simulink library "LopesDevelopmentLibrary"  (R2015b)
settings: Solver=ode45  StartTime=0.0  StopTime=10.0  RelTol=1e-3
values from neighbouring files (symbols this model uses):
  d2r = @(d) d*(pi/180)    [LopesDevelopmentLibrary_LoadParameters.m]
  ts = LopesParams.ts    [LopesDevelopmentLibrary_LoadParameters.m]
undefined symbols (not defined in the file or in its folder): anyParameterChanged, DiscIntNeverNeededParam, gcbh, LAP, LHF, LKF, LopesParams, macaddr, mxpcnetworkconfig, mxpcrtudprx, mxpcrtudptx, patientParametersChanged, port, PX, PZ, RAP, RHF, RKF, SelectorLOPESInSize, StrideTime_s, Time
undefined symbols (not defined in the file): LopesParamsSendDataArrayLen
libraries: LopesDevelopmentLibrary x327, simulink x100, dspmtrx3 x49, xpciplib x6, xpcnetworkbufferlib x5, dspsigops x4, dspstat3 x3, xpcethernetlib x2, visionstatistics x2, xpcseriallib x2, LopesDevelopmentLibraryTest x1, nmc x1
(part 3 of 12)

== system LopesDevelopmentLibrary/StringFunctions/Pad ==
  s : Inport
  pad : MATLAB Function  TreatAsAtomicUnit=on
  y : Outport
  y_len : Outport  Port=2
  wires:
  pad/1(y) -> y/1
  s/1 -> pad/1(s)
  pad/2(y_len) -> y_len/1

== system LopesDevelopmentLibrary/StringFunctions/PadStrAsDouble ==
  note: This block pads a string array; the output is as an array of doubles
      | (needed for exception blocks).
  s : Inport
  Data Type Conversion : DataTypeConversion  OutDataTypeStr=double
  pad : MATLAB Function  TreatAsAtomicUnit=on
  y : Outport
  y_len : Outport  Port=2
  wires:
  Data Type Conversion/1 -> y/1
  pad/1(y) -> Data Type Conversion/1
  s/1 -> pad/1(s)
  pad/2(y_len) -> y_len/1

== system LopesDevelopmentLibrary/StringFunctions/concat5 ==
  s1 : Inport
  s1_len : Inport  Port=2
  s2 : Inport  Port=3
  s2_len : Inport  Port=4
  s3 : Inport  Port=5
  s3_len : Inport  Port=6
  s4 : Inport  Port=7
  s4_len : Inport  Port=8
  s5 : Inport  Port=9
  s5_len : Inport  Port=10
  concat5 : MATLAB Function  TreatAsAtomicUnit=on
  str : Outport
  strLen : Outport  Port=2
  wires:
  s5_len/1 -> concat5/10(s5_len)
  s3_len/1 -> concat5/6(s3_len)
  s3/1 -> concat5/5(s3)
  concat5/1(y) -> str/1
  s1_len/1 -> concat5/2(s1_len)
  s2/1 -> concat5/3(s2)
  s4/1 -> concat5/7(s4)
  s2_len/1 -> concat5/4(s2_len)
  s4_len/1 -> concat5/8(s4_len)
  s5/1 -> concat5/9(s5)
  s1/1 -> concat5/1(s1)
  concat5/2(y_len) -> strLen/1

== system LopesDevelopmentLibrary/Various/AddToMatrixColumn ==
  A : Inport
  V : Inport  Port=2
  Maximum : Constant  Value=maximum
  Minimum : Constant  Value=minimum
  Overwrite Values : dspmtrx3/Overwrite Values  OverWriteDiag=Submatrix  valFrom2ndIP=Second input port  ConstValue=0  RowSpan=All rows  RowStartMode=Index  RowStartIndex=row  RowEndMode=Last  RowEndIndex=1  ColSpan=One column  ColStartMode=Index  ColStartIndex=col  ColEndMode=Last  ColEndIndex=1  DiagSpan=Range of elements  DiagStartMode=Index  DiagStartIndex=2  DiagEndMode=Index  DiagEndIndex=4
  Saturation Dynamic : simulink/Discontinuities/Saturation Dynamic  OutMin=[]  OutMax=[]  OutDataTypeStr=Inherit: Same as second input  OutDataType=fixdt(1, 16)  OutScaling=2^-10  DoSatur=off
  Submatrix : dspmtrx3/Submatrix  RowSpan=All rows  RowStartMode=Index  RowStartIndex=row  RowEndMode=Index  RowEndIndex=1  ColSpan=One column  ColStartMode=Index  ColStartIndex=col  ColEndMode=Last  ColEndIndex=1
  Sum : Sum  Inputs=|++
  B : Outport
  wires:
  Minimum/1 -> Saturation Dynamic/3
  Maximum/1 -> Saturation Dynamic/1
  Saturation Dynamic/1 -> Overwrite Values/2
  Sum/1 -> Saturation Dynamic/2
  A/1 -> Submatrix/1, Overwrite Values/1
  Overwrite Values/1 -> B/1
  Submatrix/1 -> Sum/1
  V/1 -> Sum/2

== system LopesDevelopmentLibrary/Various/AddToMatrixElement ==
  A : Inport
  V : Inport  Port=2
  Maximum : Constant  Value=maximum
  Minimum : Constant  Value=minimum
  Overwrite Values : dspmtrx3/Overwrite Values  OverWriteDiag=Submatrix  valFrom2ndIP=Second input port  ConstValue=0  RowSpan=One row  RowStartMode=Index  RowStartIndex=row  RowEndMode=Last  RowEndIndex=1  ColSpan=One column  ColStartMode=Index  ColStartIndex=col  ColEndMode=Last  ColEndIndex=1  DiagSpan=Range of elements  DiagStartMode=Index  DiagStartIndex=2  DiagEndMode=Index  DiagEndIndex=4
  Saturation Dynamic : simulink/Discontinuities/Saturation Dynamic  OutMin=[]  OutMax=[]  OutDataTypeStr=Inherit: Same as second input  OutDataType=fixdt(1, 16)  OutScaling=2^-10  DoSatur=off
  Submatrix : dspmtrx3/Submatrix  RowSpan=One row  RowStartMode=Index  RowStartIndex=row  RowEndMode=Index  RowEndIndex=1  ColSpan=One column  ColStartMode=Index  ColStartIndex=col  ColEndMode=Last  ColEndIndex=1
  Sum : Sum  Inputs=|++
  B : Outport
  wires:
  V/1 -> Sum/2
  Submatrix/1 -> Sum/1
  Overwrite Values/1 -> B/1
  A/1 -> Overwrite Values/1, Submatrix/1
  Sum/1 -> Saturation Dynamic/2
  Saturation Dynamic/1 -> Overwrite Values/2
  Maximum/1 -> Saturation Dynamic/1
  Minimum/1 -> Saturation Dynamic/3

== system LopesDevelopmentLibrary/Various/AdjustAmplitude ==
  note: This block multiplies all positions, velocities and accelerations by input V;
      | in other words,  it just scales the amplitude of the total curve.
  M : Inport
  V : Inport  Port=2
  Matrix Concatenate : Concatenate  Mode=Multidimensional array  ConcatenateDimension=2
  Product : Product  RndMeth=Zero
  angle_vel_acc : dspmtrx3/Submatrix  RowSpan=All rows  RowStartMode=First  RowStartIndex=1  RowEndMode=Last  RowEndIndex=1  ColSpan=Range of columns  ColStartMode=Index  ColStartIndex=2  ColEndMode=Last  ColEndIndex=1
  times : dspmtrx3/Submatrix  RowSpan=All rows  RowStartMode=First  RowStartIndex=1  RowEndMode=Last  RowEndIndex=1  ColSpan=One column  ColStartMode=First  ColStartIndex=1  ColEndMode=Last  ColEndIndex=1
  Y : Outport
  wires:
  Product/1 -> Matrix Concatenate/2
  times/1 -> Matrix Concatenate/1
  angle_vel_acc/1 -> Product/1
  Matrix Concatenate/1 -> Y/1
  M/1 -> times/1, angle_vel_acc/1
  V/1 -> Product/2

== system LopesDevelopmentLibrary/Various/AnyChanged ==
  note: Outputs true if any of the bus elements of the inputs changed during this sample.
  BusIn : Inport
  Bus to Vector : BusToVector
  Detect Change : simulink/Logic and Bit Operations/Detect Change  vinit=0  InputProcessing=Inherited  OutDataTypeStr=boolean
  Logical Operator : Logic  Operator=OR  Inputs=1  AllPortsSameDT=off  OutDataTypeStr=boolean
  Changed : Outport
  wires:
  Bus to Vector/1 -> Detect Change/1
  Detect Change/1 -> Logical Operator/1
  BusIn/1 -> Bus to Vector/1
  Logical Operator/1 -> Changed/1

== system LopesDevelopmentLibrary/Various/AssignMatrixElement ==
  A : Inport
  V : Inport  Port=2
  Maximum : Constant  Value=maximum
  Minimum : Constant  Value=minimum
  Overwrite Values : dspmtrx3/Overwrite Values  OverWriteDiag=Submatrix  valFrom2ndIP=Second input port  ConstValue=0  RowSpan=One row  RowStartMode=Index  RowStartIndex=row  RowEndMode=Last  RowEndIndex=1  ColSpan=One column  ColStartMode=Index  ColStartIndex=col  ColEndMode=Last  ColEndIndex=1  DiagSpan=Range of elements  DiagStartMode=Index  DiagStartIndex=2  DiagEndMode=Index  DiagEndIndex=4
  Saturation Dynamic : simulink/Discontinuities/Saturation Dynamic  OutMin=[]  OutMax=[]  OutDataTypeStr=Inherit: Same as second input  OutDataType=fixdt(1, 16)  OutScaling=2^-10  DoSatur=off
  B : Outport
  wires:
  Minimum/1 -> Saturation Dynamic/3
  Maximum/1 -> Saturation Dynamic/1
  Saturation Dynamic/1 -> Overwrite Values/2
  V/1 -> Saturation Dynamic/2
  Overwrite Values/1 -> B/1
  A/1 -> Overwrite Values/1

== system LopesDevelopmentLibrary/Various/BetterSpringVelocities ==
  note: If you happen to have the analytical accelerations of the spring positions,
      | you can slightly improve the performance of the system by incorporating them
      | in the velocitiy term. The idea is that the SpringVelocities_in reflect the velocity
      | at (discrete) time t=k, but they will be used throughout the sample, thus  during k<=t<k+1.
      | It would be more accurate to use the velocity halfway that period, i.e. at t=k+0.5. The best
      | estimate of that velocity we can get is by doing first order extrapolation, by using the acceleration.
      | Using Forwarrd Euler, we find v_{k+0.5} = v_k + a_k *0.5*ts, with ts the sample time.
  SpringVelocities_in : Inport
  SpringAccelerations_in : Inport  Port=2
  Add1 : Sum
  EnableAccelerationOptimization : Constant  OutDataTypeStr=double
      settings: OpenFcn=|
      | b = get_param(gcb,'value');
      | if (strcmp(b,'1')),
      |   set_param (gcb,'value','0');
      | else
      |   set_param(gcb,'value','1');
      | end;
  Half : Gain  Gain=0.5
  Product : Product  RndMeth=Zero
  SampleTimeGain : Gain  Gain=LopesParams.ts
  SpringVelocities_out : Outport
  wires:
  EnableAccelerationOptimization/1 -> Product/2
  SampleTimeGain/1 -> Half/1
  SpringAccelerations_in/1 -> SampleTimeGain/1
  Product/1 -> Add1/2
  SpringVelocities_in/1 -> Add1/1
  Add1/1 -> SpringVelocities_out/1
  Half/1 -> Product/1

== system LopesDevelopmentLibrary/Various/CompareAny ==
  In1 : Inport
  Compare To Constant : simulink/Logic and Bit Operations/Compare To Constant  relop===  const=values  OutDataTypeStr=boolean
  Logical Operator : Logic  Operator=OR  Inputs=1  AllPortsSameDT=off  OutDataTypeStr=boolean
  Out1 : Outport
  wires:
  Logical Operator/1 -> Out1/1
  Compare To Constant/1 -> Logical Operator/1
  In1/1 -> Compare To Constant/1

== system LopesDevelopmentLibrary/Various/CrossFade ==
  In1 : Inport
  In2 : Inport  Port=2
  AmountIn2 : Inport  Port=3
  Add : Sum  Inputs=+-
  Add1 : Sum
  One : Constant
  Product : Product  RndMeth=Zero
  Product1 : Product  RndMeth=Zero
  Saturation : Saturate  UpperLimit=1  LowerLimit=0
  Out : Outport
  wires:
  Add1/1 -> Out/1
  In2/1 -> Product/1
  Product1/1 -> Add1/1
  Product/1 -> Add1/2
  Add/1 -> Product1/2
  Saturation/1 -> Add/2, Product/2
  One/1 -> Add/1
  AmountIn2/1 -> Saturation/1
  In1/1 -> Product1/1

== system LopesDevelopmentLibrary/Various/CrossfadeInNSeconds ==
  note: This block cross-fades in N seconds from In1 to In2,
      | starting as soon as the block is enabled.
  note: Timer is reset on rising edge of Enable signal!
  In1 : Inport
  In2 : Inport  Port=2
  N_seconds : Inport  Port=3
  Enable : EnablePort  StatesWhenEnabling=reset
  Add : Sum
  Compare To Constant : simulink/Logic and Bit Operations/Compare To Constant  relop=>=  const=1  OutDataTypeStr=boolean
  Constant : Constant
  Counter Free-Running : simulink/Sources/Counter Free-Running  NumBits=32  tsamp=-1
  Data Type Conversion : DataTypeConversion  OutDataTypeStr=double
  Divide : Product  Inputs=*/
  Gain : Gain  Gain=LopesParams.ts
  Product : Product  RndMeth=Zero
  Product1 : Product  RndMeth=Zero
  Saturation : Saturate  UpperLimit=1  LowerLimit=0
  Subtract : Sum  Inputs=+-
  Out : Outport
  isFinished : Outport  Port=2  OutputWhenDisabled=reset  InitialOutput=[0]
  wires:
  Compare To Constant/1 -> isFinished/1
  Divide/1 -> Saturation/1, Compare To Constant/1
  N_seconds/1 -> Divide/2
  Product/1 -> Add/1
  Product1/1 -> Add/2
  Gain/1 -> Divide/1
  Counter Free-Running/1 -> Data Type Conversion/1
  Add/1 -> Out/1
  Data Type Conversion/1 -> Gain/1
  Saturation/1 -> Product1/2, Subtract/2
  In1/1 -> Product/1
  Constant/1 -> Subtract/1
  In2/1 -> Product1/1
  Subtract/1 -> Product/2

== system LopesDevelopmentLibrary/Various/Cycloid ==
  note: Given a linear input 0<=in<=1, it gives a cycloid output 0<=out<=1.
      | If In is outside the 0..1 range, it is limited to 0 or 1.
  In : Inport
  Gain1 : Gain  Gain=2*pi
  Gain2 : Gain  Gain=1/(2*pi)
  Saturation : Saturate  UpperLimit=1  LowerLimit=0
  Subtract : Sum  Inputs=+-
  Trigonometric Function : Trigonometry
  Out : Outport
  wires:
  Gain2/1 -> Subtract/2
  Trigonometric Function/1 -> Gain2/1
  Saturation/1 -> Subtract/1, Gain1/1
  In/1 -> Saturation/1
  Subtract/1 -> Out/1
  Gain1/1 -> Trigonometric Function/1

== system LopesDevelopmentLibrary/Various/Decimation ==
  note: This block outputs True  every DecimationAmount'th sample
      | (i.e., if it is 5, it will output True at sample 0, 5, 10, 15, ...).
      | If it is 1, it outputs True all the time.
  Compare To Zero : simulink/Logic and Bit Operations/Compare To Zero  relop===  OutDataTypeStr=boolean  ZeroCross=off
  Counter Free-Running : simulink/Sources/Counter Free-Running  NumBits=32  tsamp=-1
  Data Type Conversion : DataTypeConversion  OutDataTypeStr=double
  DecimationAmount : Constant  Value=Decimation
  Math Function : Math  Operator=mod  SaturateOnIntegerOverflow=on
  Decimated : Outport
  wires:
  Counter Free-Running/1 -> Data Type Conversion/1
  Data Type Conversion/1 -> Math Function/1
  Math Function/1 -> Compare To Zero/1
  DecimationAmount/1 -> Math Function/2
  Compare To Zero/1 -> Decimated/1

== system LopesDevelopmentLibrary/Various/FilteredDerivative ==
  note: This block is a derivative function
      | second order low pass filter with
      | settable zeta and omega.
      | It works for scalars as well as vectors.
      |
      | You can monitor the output from Python
      | by monitoring OutputValue.s[0,:]
  In : Inport
  Integrator : Integrator
  OutputValue : Integrator
  Product1 : Product  RndMeth=Zero
  Product2 : Product  RndMeth=Zero
  Sum : Sum  Inputs=|+-
  Sum1 : Sum  Inputs=|+-
  omega : Constant  Value=w
  omega_sq : Math  Operator=square  SaturateOnIntegerOverflow=on
  two : Constant  Value=2
  zeta : Constant  Value=z
  zeta_omega_2 : Product  Inputs=3  RndMeth=Zero
  Out : Outport
  wires:
  Product2/1 -> Sum1/2
  zeta_omega_2/1 -> Product2/2
  Product1/1 -> Sum1/1
  omega_sq/1 -> Product1/2
  zeta/1 -> zeta_omega_2/2
  two/1 -> zeta_omega_2/1
  omega/1 -> omega_sq/1, zeta_omega_2/3
  Sum/1 -> Product1/1
  OutputValue/1 -> Out/1, Integrator/1, Product2/1
  In/1 -> Sum/1
  Sum1/1 -> OutputValue/1
  Integrator/1 -> Sum/2

== system LopesDevelopmentLibrary/Various/FirstOrderLowPassFilter ==
  In : Inport
  Integrator : Integrator
  OneOverTau : Gain  Gain=1/Tau
  Sum : Sum  Inputs=|+-
  Out : Outport
  wires:
  Sum/1 -> OneOverTau/1
  Integrator/1 -> Sum/2, Out/1
  In/1 -> Sum/1
  OneOverTau/1 -> Integrator/1

== system LopesDevelopmentLibrary/Various/GenerateSyncPulseFromPhase ==
  note: This block generates a sync pulse.
      | When the phase resets (goes from 100% to 0%),
      | the sync output is set to 1 for a random time (default: between 0.1 and 0.5 s).
      | The fact that the time is random (i.e, not a repeating pattern) allows
      | for absolute syncing of two instances of the sync signal.
  Phase : Inport
  Data Type Conversion : DataTypeConversion  OutDataTypeStr=double
  DetectPhaseSignalReset : Subsystem
  GenerateRandomValue : Subsystem
  MaximumPulseLength_s : Constant  Value=0.5
  MinimumPulseLength_s : Constant  Value=0.1
  Relational Operator : RelationalOperator  Operator=<=  OutDataTypeStr=boolean
  Stopwatch : LopesLibrary/Various/Stopwatch
  SyncPulse : Outport
  wires:
  Data Type Conversion/1 -> SyncPulse/1
  Relational Operator/1 -> Data Type Conversion/1
  Stopwatch/1 -> Relational Operator/1
  GenerateRandomValue/1(Out) -> Relational Operator/2
  MinimumPulseLength_s/1 -> GenerateRandomValue/2(Minimum)
  MaximumPulseLength_s/1 -> GenerateRandomValue/1(Maximum)
  DetectPhaseSignalReset/1(PhaseReset) -> Stopwatch/1, GenerateRandomValue/Trigger
  Phase/1 -> DetectPhaseSignalReset/1(Phase)

== system LopesDevelopmentLibrary/Various/IsFirstSample ==
  note: This block outputs 1 on the first sample of the enabled block,
      | zero otherwise.
      | Note that it only works if the enable port has
      | "States when enabled" set to "reset"!
  Constant : Constant  Value=0
  Unit Delay : UnitDelay  InitialCondition=1  SampleTime=-1
  Out : Outport
  wires:
  Unit Delay/1 -> Out/1
  Constant/1 -> Unit Delay/1

== system LopesDevelopmentLibrary/Various/Latch ==
  note: Enable == HIGH: OUtput follows input
      | Enable == LOW: Output does not change anymore.
  In : Inport
  Enable : EnablePort
  Out : Outport  InitialOutput=ic
  wires:
  In/1 -> Out/1

== system LopesDevelopmentLibrary/Various/MultiplyMatrixElement ==
  A : Inport
  V : Inport  Port=2
  Maximum : Constant  Value=maximum
  Minimum : Constant  Value=minimum
  Overwrite Values : dspmtrx3/Overwrite Values  OverWriteDiag=Submatrix  valFrom2ndIP=Second input port  ConstValue=0  RowSpan=One row  RowStartMode=Index  RowStartIndex=row  RowEndMode=Last  RowEndIndex=1  ColSpan=One column  ColStartMode=Index  ColStartIndex=col  ColEndMode=Last  ColEndIndex=1  DiagSpan=Range of elements  DiagStartMode=Index  DiagStartIndex=2  DiagEndMode=Index  DiagEndIndex=4
  Product : Product  RndMeth=Zero
  Saturation Dynamic : simulink/Discontinuities/Saturation Dynamic  OutMin=[]  OutMax=[]  OutDataTypeStr=Inherit: Same as second input  OutDataType=fixdt(1, 16)  OutScaling=2^-10  DoSatur=off
  Submatrix : dspmtrx3/Submatrix  RowSpan=One row  RowStartMode=Index  RowStartIndex=row  RowEndMode=Index  RowEndIndex=1  ColSpan=One column  ColStartMode=Index  ColStartIndex=col  ColEndMode=Last  ColEndIndex=1
  B : Outport
  wires:
  Minimum/1 -> Saturation Dynamic/3
  Maximum/1 -> Saturation Dynamic/1
  Saturation Dynamic/1 -> Overwrite Values/2
  Product/1 -> Saturation Dynamic/2
  V/1 -> Product/2
  Submatrix/1 -> Product/1
  Overwrite Values/1 -> B/1
  A/1 -> Overwrite Values/1, Submatrix/1

== system LopesDevelopmentLibrary/Various/PhaseShifter1 ==
  In : Inport
  Offset_pct : Inport  Port=2
  Add : Sum
  Constant1 : Constant  Value=100
  ShiftedPhase : Math  Operator=mod  SaturateOnIntegerOverflow=on
  Out : Outport
  wires:
  Add/1 -> ShiftedPhase/1
  Offset_pct/1 -> Add/2
  In/1 -> Add/1
  ShiftedPhase/1 -> Out/1
  Constant1/1 -> ShiftedPhase/2

== system LopesDevelopmentLibrary/Various/PhaseShifter2 ==
  note: Shifts the phase by 50%
  In : Inport
  Bias : Bias  Bias=50
  Constant1 : Constant  Value=100
  ShiftedPhase : Math  Operator=mod  SaturateOnIntegerOverflow=on
  Out : Outport
  wires:
  Bias/1 -> ShiftedPhase/1
  In/1 -> Bias/1
  ShiftedPhase/1 -> Out/1
  Constant1/1 -> ShiftedPhase/2

== system LopesDevelopmentLibrary/Various/PhaseWrapper ==
  note: Wraps the input phase such
      | that the output is always
      | in the range 0<=out<100
      | (even if input is negative).
  In : Inport
  Honderd : Constant  Value=100
  ShiftedPhase1 : Math  Operator=mod  SaturateOnIntegerOverflow=on
  Out : Outport
  wires:
  ShiftedPhase1/1 -> Out/1
  In/1 -> ShiftedPhase1/1
  Honderd/1 -> ShiftedPhase1/2

== system LopesDevelopmentLibrary/Various/PhaseWrapperAroundZero ==
  note: Wraps the input phase such
      | that the output is always
      | in the range -50<=out<50.
      | This is useful for determining the difference
      | (i.e., distance) between two phase signals
  In : Inport
  Bias : Bias  Bias=50
  Honderd : Constant  Value=100
  ShiftedPhase1 : Math  Operator=mod  SaturateOnIntegerOverflow=on
  WrappedOutput : Bias  Bias=-50
  Out : Outport
  wires:
  Honderd/1 -> ShiftedPhase1/2
  In/1 -> Bias/1
  ShiftedPhase1/1 -> WrappedOutput/1
  WrappedOutput/1 -> Out/1
  Bias/1 -> ShiftedPhase1/1

== system LopesDevelopmentLibrary/Various/RateLimiterWithBypass ==
  note: If Bypass is nonzero, the rate-limiting functionality is bypassed, and the output is made equal to the input immediately.
  In : Inport
  Bypass : Inport  Port=2
  Data Type Conversion : DataTypeConversion
  IC : InitialCondition
  Rate Limiter Dynamic : simulink/Discontinuities/Rate Limiter Dynamic
  Rate_down : Constant  Value=down
  Rate_down1 : Constant  Value=-inf
  "Rate_up " : Constant  Value=up
  Rate_up1 : Constant  Value=inf
  Switch : Switch  Criteria=u2 ~= 0
  Switch1 : Switch  Criteria=u2 ~= 0
  Out : Outport
  wires:
  Data Type Conversion/1 -> IC/1
  IC/1 -> Switch1/2, Switch/2
  Rate_up1/1 -> Switch1/1
  "Rate_up "/1 -> Switch1/3
  Switch1/1 -> Rate Limiter Dynamic/1
  Switch/1 -> Rate Limiter Dynamic/3
  Rate_down/1 -> Switch/3
  Rate_down1/1 -> Switch/1
  In/1 -> Rate Limiter Dynamic/2
  Rate Limiter Dynamic/1 -> Out/1
  Bypass/1 -> Data Type Conversion/1

== system LopesDevelopmentLibrary/Various/RateLimiterWithReset ==
  u : Inport
  rate : Inport  Port=2
  initial_value : Inport  Port=3
  reset_high_active : Inport  Port=4
  RateLimiterWithReset : MATLAB Function  TreatAsAtomicUnit=on
  y : Outport
  y_is_u : Outport  Port=2
  wires:
  u/1 -> RateLimiterWithReset/1(u)
  RateLimiterWithReset/1(y) -> y/1
  rate/1 -> RateLimiterWithReset/2(rate)
  initial_value/1 -> RateLimiterWithReset/3(initialValue)
  reset_high_active/1 -> RateLimiterWithReset/4(reset_high_active)
  RateLimiterWithReset/2(y_is_u) -> y_is_u/1

== system LopesDevelopmentLibrary/Various/SLRTMessage ==
  note: This block prints the given text on the SLRT console when Trigger_in is nonzero.
      | It also relays the trigger-in signal. This way, you can put it in front of a StopSimulation
      | block and you're sure that this block is executed first.
      |
      | In its simplest form, the text-input should be a 'constant' block, with as value something like:
      | uint8('This message is printed')
  Trigger_in : Inport
  Text : Inport  Port=2
  Data Type Conversion : DataTypeConversion
  Data Type Conversion1 : DataTypeConversion
  Pad : LopesDevelopmentLibrary/StringFunctions/Pad  outArrayLen=200
  S-Function Builder : S-Function  InitFcn=try, set_param(gcb,'FunctionName','SLRTMessage'), end  FunctionName=SLRTMessage  SFunctionModules=SLRTMessage_wrapper  SFunctionDeploymentMode=off  EnableBusSupport=off  mask(S-Function Builder){}
      mask help: Simulink:masks:SFunctionBuilder_MD
      mask init:
      | val = [[.9  0.75 0.75 1 1 .9 .9 1]',[1 1 0.75 0.75 .9 .9 1 .9]'];try , sys = get_param(gcb,'SfunBuilderFcnName');if isempty(sys), sys = get_param(gcb,'FunctionName'); end,catch, sys = get_param(gcb,'FunctionName'); end
      settings: CopyFcn=set_param(gcbh,'LinkStatus','none')  PreSaveFcn=try, set_param(gcb,'FunctionName','SLRTMessage'), end  OpenFcn=sfunctionwizard(gcbh)
      mask Display: plot(val(:,1),val(:,2)),disp(sys), port_label('input',1,'trigger'), port_label('input',2,'text'), port_label('output',1,'trigger_out')
  Terminator : Terminator
  Trigger_out : Outport
  wires:
  Pad/2 -> Terminator/1
  Data Type Conversion/1 -> S-Function Builder/1
  S-Function Builder/1 -> Data Type Conversion1/1
  Text/1 -> Pad/1
  Pad/1 -> S-Function Builder/2
  Trigger_in/1 -> Data Type Conversion/1
  Data Type Conversion1/1 -> Trigger_out/1

== system LopesDevelopmentLibrary/Various/SafeDivide ==
  note: This block guarantees division-by-zero-free division.
  Numerator : Inport
  Denominator : Inport  Port=2
  Add : Sum
  Compare To Zero : simulink/Logic and Bit Operations/Compare To Zero  relop===  OutDataTypeStr=boolean
  Data Type Conversion : DataTypeConversion  OutDataTypeStr=double
  Divide : Product  Inputs=*/
  Gain1 : Gain  Gain=1e-100
  Out : Outport
  wires:
  Data Type Conversion/1 -> Gain1/1
  Gain1/1 -> Add/2
  Add/1 -> Divide/2
  Denominator/1 -> Compare To Zero/1, Add/1
  Numerator/1 -> Divide/1
  Divide/1 -> Out/1
  Compare To Zero/1 -> Data Type Conversion/1

== system LopesDevelopmentLibrary/Various/Sample Number Generator ==
  note: Sample Number Generator
      |
      | Put this block once somewhere
      | (preferably in the main window).
      | Then, use the SampleNumber
      | block from the LopesDevelopmentLibrary
      | (in sublibrary Various) to get the
      | sample number.
      | Advantage of using this instead of a
      | free running counter and converter
      | every time you need the sample
      | number:  the sample number is
      | only calculated once, and that disabling blocks
      | does not cause the sample number to freeze.
      |
      | Note: You need to put a DataStore block with
      | identifier SAMPLENO in the main window.
  Counter Free-Running : simulink/Sources/Counter Free-Running  NumBits=32  tsamp=-1
  Data Store Write : DataStoreWrite  DataStoreName=SAMPLENO
  Data Type Conversion : DataTypeConversion  OutDataTypeStr=double
  wires:
  Data Type Conversion/1 -> Data Store Write/1
  Counter Free-Running/1 -> Data Type Conversion/1

== system LopesDevelopmentLibrary/Various/SampleNumber ==
  note: This block outputs the sample number
      | as a double.
  Data Store Read : DataStoreRead  DataStoreName=SAMPLENO  SampleTime=LopesParams.ts
  SampleNumber : Outport
  wires:
  Data Store Read/1 -> SampleNumber/1

== system LopesDevelopmentLibrary/Various/SecondOrderHighPassFilter ==
  note: This is an implementation of a
      | second order high pass filter with
      | settable zeta and omega.
      | It works for scalars as well as vectors.
      |
      | You can monitor the output from Python
      | by monitoring OutputValue.s[0,:]
  In : Inport
  Integrator : Integrator
  Integrator2 : Integrator
  OutputValue : Sum  Inputs=-+
  Product1 : Product  RndMeth=Zero
  Product2 : Product  RndMeth=Zero
  Sum : Sum  Inputs=|+-
  Sum1 : Sum  Inputs=|+-
  omega : Constant  Value=w
  omega_sq : Math  Operator=square  SaturateOnIntegerOverflow=on
  two : Constant  Value=2
  zeta : Constant  Value=z
  zeta_omega_2 : Product  Inputs=3  RndMeth=Zero
  Out : Outport
  wires:
  Product2/1 -> Sum1/2
  zeta_omega_2/1 -> Product2/2
  Product1/1 -> Sum1/1
  omega_sq/1 -> Product1/2
  zeta/1 -> zeta_omega_2/2
  two/1 -> zeta_omega_2/1
  omega/1 -> omega_sq/1, zeta_omega_2/3
  Sum/1 -> Product1/1
  Integrator/1 -> Integrator2/1, Product2/1
  In/1 -> OutputValue/2, Sum/1
  Sum1/1 -> Integrator/1
  Integrator2/1 -> OutputValue/1, Sum/2
  OutputValue/1 -> Out/1

== system LopesDevelopmentLibrary/Various/SecondOrderLowPassFilter ==
  note: This is an implementation of a
      | second order low pass filter with
      | settable zeta and omega.
      | It works for scalars as well as vectors.
      |
      | You can monitor the output from Python
      | by monitoring OutputValue.s[0,:]
  In : Inport
  Integrator : Integrator
  OutputValue : Integrator
  Product1 : Product  RndMeth=Zero
  Product2 : Product  RndMeth=Zero
  Sum : Sum  Inputs=|+-
  Sum1 : Sum  Inputs=|+-
  omega : Constant  Value=w
  omega_sq : Math  Operator=square  SaturateOnIntegerOverflow=on
  two : Constant  Value=2
  zeta : Constant  Value=z
  zeta_omega_2 : Product  Inputs=3  RndMeth=Zero
  Out : Outport
  wires:
  OutputValue/1 -> Out/1, Sum/2
  Sum1/1 -> Integrator/1
  In/1 -> Sum/1
  Integrator/1 -> Product2/1, OutputValue/1
  Sum/1 -> Product1/1
  omega/1 -> zeta_omega_2/3, omega_sq/1
  two/1 -> zeta_omega_2/1
  zeta/1 -> zeta_omega_2/2
  omega_sq/1 -> Product1/2
  Product1/1 -> Sum1/1
  zeta_omega_2/1 -> Product2/2
  Product2/1 -> Sum1/2

== system LopesDevelopmentLibrary/Various/Split ==
  note: Thsi block splits up an 13-element vector (containing info
      | of both actuated and unactuated joints) into two
      | parts: the actuated (10-element) and unactauted (3-element) part.
  Input : Inport
  Actuated1 : Selector  InputPortWidth=13  IndexOptions=Index vector (dialog)  Indices=1:10  OutputSizes=1
  Unactuated1 : Selector  InputPortWidth=13  IndexOptions=Index vector (dialog)  Indices=11:13  OutputSizes=1
  Actuated : Outport
  Unactuated : Outport  Port=2
  wires:
  Unactuated1/1 -> Unactuated/1
  Actuated1/1 -> Actuated/1
  Input/1 -> Actuated1/1, Unactuated1/1

== system LopesDevelopmentLibrary/Various/Stopwatch ==
  note: Stopwatch -
      | Outputs time in seconds.
      | Reset during high level of Rest pulse
  ResetHighActive : Inport
  Counter Free-Running : simulink/Sources/Counter Free-Running  NumBits=32  tsamp=-1
  Data Type Conversion : DataTypeConversion  OutDataTypeStr=double
  Gain : Gain  Gain=LopesParams.ts
  Latch : LopesDevelopmentLibrary/Various/Latch  ic=0
  Subtract : Sum  Inputs=+-
  Time_s : Outport
  wires:
  ResetHighActive/1 -> Latch/Enable
  Data Type Conversion/1 -> Gain/1
  Gain/1 -> Time_s/1
  Latch/1 -> Subtract/2  "startTime"
  Subtract/1 -> Data Type Conversion/1
  Counter Free-Running/1 -> Subtract/1, Latch/1

== system LopesDevelopmentLibrary/Various/TriggerAtPhaseCrossing ==
  Phase : Inport
  PhaseToTrigger : Inport  Port=2
  Detect Rise Nonnegative : simulink/Logic and Bit Operations/Detect Rise Nonnegative  vinit=0  InputProcessing=Inherited  OutDataTypeStr=boolean
  PhaseWrapperAroundZero : LopesDevelopmentLibrary/Various/PhaseWrapperAroundZero
  Subtract : Sum  Inputs=+-
  Trigger : Outport
  wires:
  Detect Rise Nonnegative/1 -> Trigger/1
  Phase/1 -> Subtract/1
  Subtract/1 -> PhaseWrapperAroundZero/1
  PhaseToTrigger/1 -> Subtract/2
  PhaseWrapperAroundZero/1 -> Detect Rise Nonnegative/1

== system LopesDevelopmentLibrary/Various/WeightedAverage ==
  note: This block takes the 'weighted average' of inputs In0 and In1.
      | The weighing factor is set by the Ratio input, eg:
      | Ratio=0 -> Take input 0
      | Ratio=0.4 -> Take 0.6*input0  + 0.4*input1
      | Ratio=1 -> Take input1
      | General: Output = (1-Ratio)*input0 + Ratio*input1
  In0 : Inport
  In1 : Inport  Port=2
  Ratio : Inport  Port=3
  Multiply0 : Product  Inputs=**
  Multiply1 : Product  Inputs=**
  One : Constant
  Saturation : Saturate  UpperLimit=1  LowerLimit=0
  Subtract : Sum  Inputs=+-
  Sum : Sum
  Out : Outport
  wires:
  Ratio/1 -> Saturation/1
  In1/1 -> Multiply1/1
  Multiply1/1 -> Sum/2
  Subtract/1 -> Multiply0/2
  Saturation/1 -> Multiply1/2, Subtract/2
  Sum/1 -> Out/1
  Multiply0/1 -> Sum/1
  One/1 -> Subtract/1
  In0/1 -> Multiply0/1

== system LopesDevelopmentLibrary/BlocksForInternalUse/GaitGeneration/CalculateCartesianPositions ==
  note: Input for s-function,
      | jointAngles:
      | PelvisPosX
      | PelvixPosY
      | PelvisPosZ
      | PelvisAxialAngle
      | PelvisFrontalAngle
      | LHA
      | LHF
      | LHEndorotatoin
      | LKF
      | LAEndorotation
      | LAP
      | LAInversion
      | RHA
      | RHF
      | RHEnorotation
      | RKF
      | RAEndorotation
      | RAP
      | RAInversion
  note: Input for s-function,
      | patientDimensions:
      | Mass
      | BodyLength
      | PelvisWidth
      | PelvisHeight
      | ThighLeftLength
      | ThighRightLength
      | ShankLeftLength
      | ShankRightLength
      | FootLeftLength
      | FootRightLength
      | FootLeftHeight
      | FootRightHeight
  Parameters : Inport
  jointAngles : Inport  Port=2
  forceOneFootOnGround : Inport  Port=3
  ConvertFromAnkleAnglesToFootAngles : Subsystem
  ExtractPatientParameters : Subsystem
  OmitAnklesAndToes : Subsystem
  S-Function : S-Function  FunctionName=KinHuman_sfunction  SFunctionModules='KinHuman KinObject KinPointAxis KinHuman_common'  SFunctionDeploymentMode=off  EnableBusSupport=off
      mask Display:
      | port_label('input',1,'patientDimensions')
      | port_label('input',2,'patientDimensionsChanged')
      | port_label('input',3,'jointAngles')
      | port_label('input',4,'forceOneFootOnGround')
      | port_label('output',1,'CartesianPositions')
      | port_label('output',2,'PY')
  CartesianPositions : Outport
  PY_new : Outport  Port=2  OutDataTypeStr=double
  wires:
  Parameters/1 -> ExtractPatientParameters/1(Parameters)
  ConvertFromAnkleAnglesToFootAngles/1(Out) -> S-Function/3
  jointAngles/1 -> ConvertFromAnkleAnglesToFootAngles/1(In)
  OmitAnklesAndToes/1(Out) -> CartesianPositions/1
  S-Function/1 -> OmitAnklesAndToes/1(In)
  forceOneFootOnGround/1 -> S-Function/4
  ExtractPatientParameters/1(PatientDimensions) -> S-Function/1
  ExtractPatientParameters/2(DimensionsChanged) -> S-Function/2
  S-Function/2 -> PY_new/1

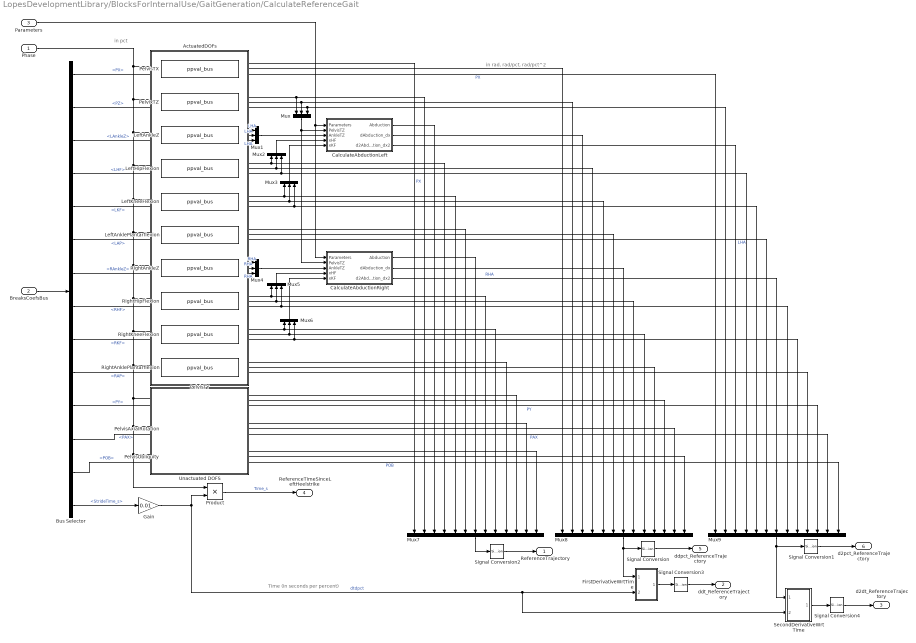
== system LopesDevelopmentLibrary/BlocksForInternalUse/GaitGeneration/CalculateReferenceGait ==
  note: Time (in seconds per percent)
  note: in rad, rad/pct, rad/pct^2
  note: in pct
  Phase : Inport
  BreaksCoefsBus : Inport  Port=2
  Parameters : Inport  Port=3
  ActuatedDOFs : Subsystem
      mask Display: disp('')
  Bus Selector : BusSelector  OutputSignals=PX,PZ,LAnkleZ,LHF,LKF,LAP,RAnkleZ,RHF,RKF,RAP,PY,PAX,POB,StrideTime_s
  CalculateAbductionLeft : Subsystem  mask{isRight=0}
      mask prompts: isRight "Is Right Leg"
  CalculateAbductionRight : Subsystem  mask{isRight=1}
      mask prompts: isRight "Is Right Leg"
  FirstDerivativeWrtTime : Subsystem
  Gain : Gain  Gain=0.01
  LeftAnklePlantarflexion : LopesDevelopmentLibrary/BlocksForInternalUse/GaitGeneration/ppval_bus
  LeftAnkleZ : LopesDevelopmentLibrary/BlocksForInternalUse/GaitGeneration/ppval_bus
  LeftHipFlexion : LopesDevelopmentLibrary/BlocksForInternalUse/GaitGeneration/ppval_bus
  LeftKneeFlexion : LopesDevelopmentLibrary/BlocksForInternalUse/GaitGeneration/ppval_bus
  Mux{,1..6} (7 alike) : Mux  Inputs=3
  Mux7 : Mux  Inputs=13
  Mux8 : Mux  Inputs=13
  Mux9 : Mux  Inputs=13
  PelvisAxialRotation : LopesDevelopmentLibrary/BlocksForInternalUse/GaitGeneration/ppval_bus
  PelvisObliquity : LopesDevelopmentLibrary/BlocksForInternalUse/GaitGeneration/ppval_bus
  PelvisTX : LopesDevelopmentLibrary/BlocksForInternalUse/GaitGeneration/ppval_bus
  PelvisTY : LopesDevelopmentLibrary/BlocksForInternalUse/GaitGeneration/ppval_bus
  PelvixTZ : LopesDevelopmentLibrary/BlocksForInternalUse/GaitGeneration/ppval_bus
  Product : Product  RndMeth=Zero
  RightAnklePlantarflexion : LopesDevelopmentLibrary/BlocksForInternalUse/GaitGeneration/ppval_bus
  RightAnkleZ : LopesDevelopmentLibrary/BlocksForInternalUse/GaitGeneration/ppval_bus
  RightHipFlexion : LopesDevelopmentLibrary/BlocksForInternalUse/GaitGeneration/ppval_bus
  RightKneeFlexion : LopesDevelopmentLibrary/BlocksForInternalUse/GaitGeneration/ppval_bus
  SecondDerivativeWrtTime : Subsystem
  Signal Conversion{,1..4} (5 alike) : SignalConversion
  Unactuated DOFS : Subsystem
      mask Display: disp('')
  ReferenceTrajectory : Outport
  ddt_ReferenceTrajectory : Outport  Port=2
  d2dt_ReferenceTrajectory : Outport  Port=3
  ReferenceTimeSinceLeftHeelstrike : Outport  Port=4
  ddpct_ReferenceTrajectory : Outport  Port=5
  d2pct_ReferenceTrajectory : Outport  Port=6
  wires:
  RightAnklePlantarflexion/3 -> Mux9/10
  RightAnklePlantarflexion/2 -> Mux8/10
  LeftAnklePlantarflexion/3 -> Mux9/6
  LeftAnklePlantarflexion/2 -> Mux8/6
  RightAnklePlantarflexion/1 -> Mux7/10
  LeftAnklePlantarflexion/1 -> Mux7/6
  Bus Selector/10 -> RightAnklePlantarflexion/2  "<RAP>"
  Bus Selector/6 -> LeftAnklePlantarflexion/2  "<LAP>"
  PelvisObliquity/3 -> Mux9/13  "POB"
  PelvisAxialRotation/3 -> Mux9/12  "PAX"
  PelvisTY/3 -> Mux9/11  "PY"
  CalculateAbductionRight/3(d2Abduction_dx2) -> Mux9/7  "RHA"
  CalculateAbductionLeft/3(d2Abduction_dx2) -> Mux9/3  "LHA"
  PelvisTX/3 -> Mux9/1  "PX"
  Mux7/1 -> Signal Conversion2/1
  PelvisTX/1 -> Mux7/1  "PX"
  Mux5/1 -> CalculateAbductionRight/4(xHF)
  Mux6/1 -> CalculateAbductionRight/5(xKF)
  Mux4/1 -> CalculateAbductionRight/3(AnkleTZ)
  RightAnkleZ/1 -> Mux4/1  "RHA"
  RightAnkleZ/3 -> Mux4/3  "RHA"
  RightAnkleZ/2 -> Mux4/2  "RHA"
  Mux3/1 -> CalculateAbductionLeft/5(xKF)
  Mux2/1 -> CalculateAbductionLeft/4(xHF)
  Mux1/1 -> CalculateAbductionLeft/3(AnkleTZ)
  Mux/1 -> CalculateAbductionLeft/2(PelvisTZ), CalculateAbductionRight/2(PelvisTZ)
  Signal Conversion4/1 -> d2dt_ReferenceTrajectory/1
  Signal Conversion3/1 -> ddt_ReferenceTrajectory/1
  Signal Conversion2/1 -> ReferenceTrajectory/1
  Signal Conversion1/1 -> d2pct_ReferenceTrajectory/1
  Signal Conversion/1 -> ddpct_ReferenceTrajectory/1
  LeftAnkleZ/3 -> Mux1/3  "LHA"
  LeftAnkleZ/2 -> Mux1/2  "LHA"
  LeftAnkleZ/1 -> Mux1/1  "LHA"
  Parameters/1 -> CalculateAbductionLeft/1(Parameters), CalculateAbductionRight/1(Parameters)
  PelvisTY/2 -> Mux8/11
  PelvisTY/1 -> Mux7/11
  PelvisObliquity/1 -> Mux7/13
  LeftHipFlexion/1 -> Mux2/1, Mux7/4
  PelvixTZ/1 -> Mux/1, Mux7/2
  Bus Selector/9 -> RightKneeFlexion/2  "<RKF>"
  Phase/1 -> RightAnkleZ/1, RightHipFlexion/1, RightKneeFlexion/1, PelvisTY/1, PelvisAxialRotation/1, PelvisObliquity/1, Product/1, RightAnklePlantarflexion/1, LeftAnklePlantarflexion/1, LeftKneeFlexion/1, LeftHipFlexion/1, LeftAnkleZ/1, PelvixTZ/1, PelvisTX/1
  LeftKneeFlexion/1 -> Mux3/1, Mux7/5
  PelvisTX/2 -> Mux8/1
  PelvixTZ/2 -> Mux/2, Mux8/2
  RightKneeFlexion/1 -> Mux6/1, Mux7/9
  RightHipFlexion/1 -> Mux5/1, Mux7/8
  CalculateAbductionLeft/2(dAbduction_dx) -> Mux8/3
  LeftHipFlexion/2 -> Mux2/2, Mux8/4
  LeftKneeFlexion/2 -> Mux3/2, Mux8/5
  RightHipFlexion/2 -> Mux5/2, Mux8/8
  Mux9/1 -> Signal Conversion1/1, SecondDerivativeWrtTime/1(ddydx)
  PelvixTZ/3 -> Mux/3, Mux9/2
  RightKneeFlexion/3 -> Mux6/3, Mux9/9
  Bus Selector/14 -> Gain/1  "<StrideTime_s>"
  PelvisAxialRotation/1 -> Mux7/12
  Product/1 -> ReferenceTimeSinceLeftHeelstrike/1  "Time_s"
  FirstDerivativeWrtTime/1(dydt) -> Signal Conversion3/1
  SecondDerivativeWrtTime/1(ddydt) -> Signal Conversion4/1
  PelvisObliquity/2 -> Mux8/13
  PelvisAxialRotation/2 -> Mux8/12
  Bus Selector/13 -> PelvisObliquity/2  "<POB>"
  Bus Selector/12 -> PelvisAxialRotation/2  "<PAX>"
  Bus Selector/11 -> PelvisTY/2  "<PY>"
  Mux8/1 -> FirstDerivativeWrtTime/1(dydx), Signal Conversion/1
  Gain/1 -> FirstDerivativeWrtTime/2(dtdx), SecondDerivativeWrtTime/2(dtdx), Product/2  "dtdpct"
  BreaksCoefsBus/1 -> Bus Selector/1
  Bus Selector/2 -> PelvixTZ/2  "<PZ>"
  Bus Selector/1 -> PelvisTX/2  "<PX>"
  Bus Selector/4 -> LeftHipFlexion/2  "<LHF>"
  Bus Selector/8 -> RightHipFlexion/2  "<RHF>"
  Bus Selector/3 -> LeftAnkleZ/2  "<LAnkleZ>"
  Bus Selector/7 -> RightAnkleZ/2  "<RAnkleZ>"
  Bus Selector/5 -> LeftKneeFlexion/2  "<LKF>"
  CalculateAbductionLeft/1(Abduction) -> Mux7/3
  CalculateAbductionRight/1(Abduction) -> Mux7/7
  CalculateAbductionRight/2(dAbduction_dx) -> Mux8/7
  RightKneeFlexion/2 -> Mux6/2, Mux8/9
  LeftHipFlexion/3 -> Mux2/3, Mux9/4
  LeftKneeFlexion/3 -> Mux3/3, Mux9/5
  RightHipFlexion/3 -> Mux5/3, Mux9/8

== system LopesDevelopmentLibrary/BlocksForInternalUse/GaitGeneration/CalculateStiffnessForOneJoint ==
  note: \beta_{j,m}(phi)
  note: y_{j,m}(phi)
  note: See LopesTechnicalDocumentation
  GeneralStiffness_pct : Inport
  AspectAlphas : Inport  Port=2
  AspectStiffnesses : Inport  Port=3
  Abs : Abs
  Add : Sum
  AvoidDivisionByZero : Bias  Bias=1e-10
  CalculateDenominator : Sum  Inputs=+
  CalculateNumerator : Sum  Inputs=+
  Divide : Product  Inputs=*/
  NumeratorElements : Product  RndMeth=Zero
  Product : Product  RndMeth=Zero
  Subtract : Sum  Inputs=+-
  Stiffness_pct : Outport
  wires:
  CalculateNumerator/1 -> Divide/1
  CalculateDenominator/1 -> AvoidDivisionByZero/1
  Divide/1 -> Add/1
  AvoidDivisionByZero/1 -> Divide/2
  NumeratorElements/1 -> CalculateNumerator/1
  Abs/1 -> NumeratorElements/2, CalculateDenominator/1
  Product/1 -> Abs/1, NumeratorElements/1
  AspectAlphas/1 -> Product/1
  Subtract/1 -> Product/2
  AspectStiffnesses/1 -> Subtract/1
  GeneralStiffness_pct/1 -> Subtract/2, Add/2
  Add/1 -> Stiffness_pct/1

== system LopesDevelopmentLibrary/BlocksForInternalUse/GaitGeneration/OrderKeyEvents ==
  kE : Inport
  JointNumber : Inport  Port=2
  SortKeyEvents : MATLAB Function  TreatAsAtomicUnit=on
  kE_out : Outport
  isError : Outport  Port=2
  wires:
  SortKeyEvents/1(kE_out) -> kE_out/1
  SortKeyEvents/2(Error) -> isError/1
  kE/1 -> SortKeyEvents/1(kE)
  JointNumber/1 -> SortKeyEvents/2(jointNumber)

== system LopesDevelopmentLibrary/BlocksForInternalUse/GaitGeneration/RegressionData2KeyEvents ==
  regressionParameters : Inport
  parameters : Inport  Port=2
  Bus Selector : BusSelector  OutputSignals=General.WalkingVelocity_m_s,Patient.BodyLength_m
  RegressionData2KeyEvents : MATLAB Function  TreatAsAtomicUnit=on
  keyEvents : Outport
  wires:
  Bus Selector/2 -> RegressionData2KeyEvents/3(bodyLength)  "<BodyLength_m>"
  Bus Selector/1 -> RegressionData2KeyEvents/2(v)  "<WalkingVelocity_m_s>"
  parameters/1 -> Bus Selector/1
  RegressionData2KeyEvents/1(keyEvents) -> keyEvents/1
  regressionParameters/1 -> RegressionData2KeyEvents/1(regressionParameters)

== system LopesDevelopmentLibrary/BlocksForInternalUse/GaitGeneration/SmoothlyRemove2ndKE ==
  KE_in : Inport
  v : Inport  Port=2
  SmoothlyRemoveSecondKeyEvent : MATLAB Function  TreatAsAtomicUnit=on
  KE_out : Outport
  wires:
  SmoothlyRemoveSecondKeyEvent/1(KE_out) -> KE_out/1
  v/1 -> SmoothlyRemoveSecondKeyEvent/2(v)
  KE_in/1 -> SmoothlyRemoveSecondKeyEvent/1(KE_in)

== system LopesDevelopmentLibrary/BlocksForInternalUse/GaitGeneration/TrajectoryOfInfluence ==
  TrajectoryOfInfluenceParameters : Inport
  keyEventTimes : Inport  Port=2
  phase : Inport  Port=3
  TrajectoryOfInfluence : MATLAB Function  TreatAsAtomicUnit=on
  alpha : Outport
  wires:
  phase/1 -> TrajectoryOfInfluence/3(phase)
  TrajectoryOfInfluenceParameters/1 -> TrajectoryOfInfluence/1(parameters)
  TrajectoryOfInfluence/1(alpha) -> alpha/1
  keyEventTimes/1 -> TrajectoryOfInfluence/2(keyEventTimes)

== system LopesDevelopmentLibrary/BlocksForInternalUse/GaitGeneration/keyEvents2breakscoefs3 ==
  keyEvents : Inport
  keyEvents2breakscoefs3 : MATLAB Function  TreatAsAtomicUnit=on
  breaks : Outport
  coefs : Outport  Port=2
  wires:
  keyEvents2breakscoefs3/2(coefs) -> coefs/1
  keyEvents/1 -> keyEvents2breakscoefs3/1(keyEvents)
  keyEvents2breakscoefs3/1(breaks) -> breaks/1

== system LopesDevelopmentLibrary/BlocksForInternalUse/GaitGeneration/keyEvents2breakscoefs5 ==
  keyEvents : Inport
  keyEvents2breakscoefs5 : MATLAB Function  TreatAsAtomicUnit=on
  breaks : Outport
  coefs : Outport  Port=2
  wires:
  keyEvents2breakscoefs5/1(breaks) -> breaks/1
  keyEvents/1 -> keyEvents2breakscoefs5/1(keyEvents)
  keyEvents2breakscoefs5/2(coefs) -> coefs/1

== system LopesDevelopmentLibrary/BlocksForInternalUse/GaitGeneration/ppval_bus ==
  xx : Inport
  BreaksCoefs : Inport  Port=2
  Bus Selector1 : BusSelector  OutputSignals=breaks,coefs
  ppval : MATLAB Function  TreatAsAtomicUnit=on
  yy : Outport
  dydx : Outport  Port=2
  ddydx : Outport  Port=3
  wires:
  Bus Selector1/1 -> ppval/2(breaks)  "<breaks>"
  Bus Selector1/2 -> ppval/3(coefs)  "<coefs>"
  xx/1 -> ppval/1(xx)
  BreaksCoefs/1 -> Bus Selector1/1
  ppval/1(yy) -> yy/1
  ppval/2(dydx) -> dydx/1
  ppval/3(ddydx) -> ddydx/1

== system LopesDevelopmentLibrary/BlocksForInternalUse/GaitGenerationStartStop/AddUselessKE ==
  kE : Inport
  BreaksCoefs : Inport  Port=2
  AddUselessKE : MATLAB Function  TreatAsAtomicUnit=on
  Bus Selector1 : BusSelector  OutputSignals=breaks
  kE_out : Outport
  wires:
  Bus Selector1/1 -> AddUselessKE/2(breaks)  "<breaks>"
  kE/1 -> AddUselessKE/1(kE)
  AddUselessKE/1(kE_out) -> kE_out/1
  BreaksCoefs/1 -> Bus Selector1/1

== system LopesDevelopmentLibrary/BlocksForInternalUse/GaitGenerationStartStop/AddUselessKEValue ==
  note: This is needed because the Startup/SlowDown SubSystem has more key events
      | Bus signals require to be te same size
  kE : Inport
  AddUselessKE : MATLAB Function  TreatAsAtomicUnit=on
  kE_out : Outport
  wires:
  AddUselessKE/1(kE_out) -> kE_out/1
  kE/1 -> AddUselessKE/1(kE)

== system LopesDevelopmentLibrary/BlocksForInternalUse/GaitGenerationStartStop/CalculateKEforStartup ==
  kE : Inport
  BreaksCoefsForThisJoint : Inport  Port=2
  JointNumber : Inport  Port=3
  ConnectionPoint : Inport  Port=4
  AddUselessKE : LopesDevelopmentLibrary/BlocksForInternalUse/GaitGenerationStartStop/AddUselessKE
  CalcKe : LopesDevelopmentLibrary/BlocksForInternalUse/GaitGeneration/ppval_bus
  OrderKeyEventsAddOne : LopesDevelopmentLibrary/BlocksForInternalUse/GaitGenerationStartStop/OrderKeyEventsAddOne
  Terminator : Terminator
  kE_out : Outport
  Error : Outport  Port=2
  wires:
  JointNumber/1 -> OrderKeyEventsAddOne/2
  kE/1 -> OrderKeyEventsAddOne/1
  BreaksCoefsForThisJoint/1 -> CalcKe/2, AddUselessKE/2
  ConnectionPoint/1 -> OrderKeyEventsAddOne/3, CalcKe/1
  CalcKe/3 -> Terminator/1
  CalcKe/2 -> OrderKeyEventsAddOne/5
  CalcKe/1 -> OrderKeyEventsAddOne/4
  AddUselessKE/1 -> kE_out/1
  OrderKeyEventsAddOne/2 -> Error/1
  OrderKeyEventsAddOne/1 -> AddUselessKE/1
